simulink model "covid"  (R2019b)
settings: Solver=ode23s  StartTime=0.0  StopTime=50  FixedStep=1
values from neighbouring files (symbols this model uses):
  optimprob = optim.openProblem(Country, Province)    [main.m]
undefined symbols (not defined in the file or in its folder): D0, E0, I0, P0, Q0, R0, S0, x
settings Model: SimulationMode=accelerator  OrderedModelArguments=off  Creator=SaDiablo  LastModifiedBy=SaDiablo
settings SolverCC: MaxConsecutiveMinStep=1e4  ZeroCrossAlgorithm=Adaptive
settings DataIOCC: SaveState=on
settings DebuggingCC: MaxConsecutiveZCsMsg=warning  MaskedZcDiagnostic=none
settings HardwareCC: ProdHWDeviceType=AMD->x86-64 (Windows64)

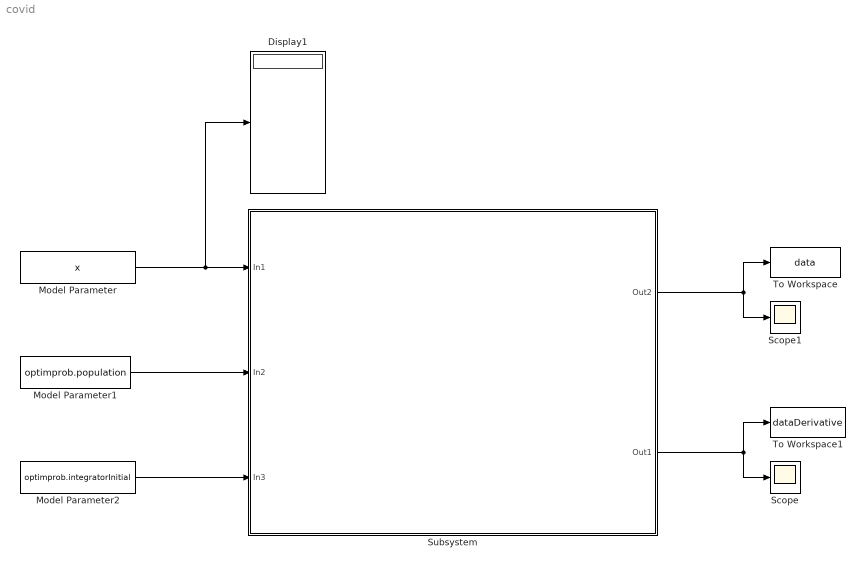
== system covid ==
  Display1 : Display
  Model Parameter : Constant  Value=x
  Model Parameter1 : Constant  Value=optimprob.population
  Model Parameter2 : Constant  Value=optimprob.integratorInitial
  Scope : Scope
  Scope1 : Scope
  Subsystem : Subsystem
  To Workspace : ToWorkspace  VariableName=data  SaveFormat=Timeseries  SampleTime=-1
  To Workspace1 : ToWorkspace  VariableName=dataDerivative  SaveFormat=Timeseries  SampleTime=-1
  wires:
  Model Parameter/1 -> Subsystem/1(In1), Display1/1
  Subsystem/1(Out2) -> Scope1/1, To Workspace/1
  Subsystem/2(Out1) -> Scope/1, To Workspace1/1
  Model Parameter2/1 -> Subsystem/3(In3)
  Model Parameter1/1 -> Subsystem/2(In2)

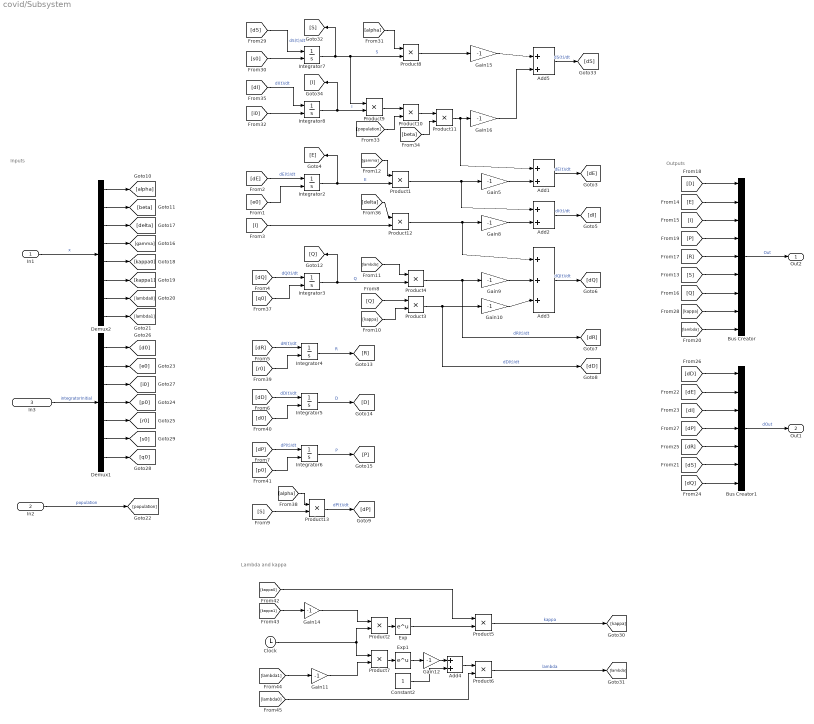
== system covid/Subsystem ==
  note: Inputs
  note: Outputs
  note: Lambda and kappa
  In1 : Inport
  In2 : Inport  Port=2
  In3 : Inport  Port=3
  Add1 : Sum  Inputs=+|+
  Add2 : Sum  Inputs=+|+
  Add3 : Sum  Inputs=+|+|+
  Add4 : Sum
  Add5 : Sum  Inputs=+|+
  Bus Creator : BusCreator  Inputs=9
  Bus Creator1 : BusCreator  Inputs=7
  Clock : Clock
  Constant2 : Constant
  Demux1 : Demux  Outputs=7
  Demux2 : Demux  Outputs=8
  Exp : Math  SignedPower=off  SaturateOnIntegerOverflow=on
  Exp1 : Math  SignedPower=off  SaturateOnIntegerOverflow=on
  Gain{5,8..12,14..16} (9 alike) : Gain  Gain=-1
  Integrator2 : Integrator  InitialConditionSource=external  InitialCondition=E0  LimitOutput=on  UpperSaturationLimit=optimprob.population  LowerSaturationLimit=0  WrappedStateUpperValue=population  WrappedStateLowerValue=0  ZeroCross=off  ContinuousStateAttributes='E'
  Integrator3 : Integrator  InitialConditionSource=external  InitialCondition=Q0  LimitOutput=on  UpperSaturationLimit=optimprob.population  LowerSaturationLimit=0  WrappedStateUpperValue=population  WrappedStateLowerValue=0  ZeroCross=off
  Integrator4 : Integrator  InitialConditionSource=external  InitialCondition=R0  LimitOutput=on  UpperSaturationLimit=optimprob.population  LowerSaturationLimit=0  WrappedStateUpperValue=population  WrappedStateLowerValue=0
  Integrator5 : Integrator  InitialConditionSource=external  InitialCondition=D0  LimitOutput=on  UpperSaturationLimit=optimprob.population  LowerSaturationLimit=0  WrappedStateUpperValue=population  WrappedStateLowerValue=0
  Integrator6 : Integrator  InitialConditionSource=external  InitialCondition=P0  LimitOutput=on  UpperSaturationLimit=optimprob.population  LowerSaturationLimit=0  WrappedStateUpperValue=population  WrappedStateLowerValue=0
  Integrator7 : Integrator  InitialConditionSource=external  InitialCondition=S0  LimitOutput=on  UpperSaturationLimit=optimprob.population  LowerSaturationLimit=0  WrappedStateUpperValue=population  WrappedStateLowerValue=0  ZeroCross=off
  Integrator8 : Integrator  InitialConditionSource=external  InitialCondition=I0  LimitOutput=on  UpperSaturationLimit=optimprob.population  LowerSaturationLimit=0  WrappedStateUpperValue=population  WrappedStateLowerValue=0  ZeroCross=off
  Product{1..13} (13 alike) : Product
  Out2 : Outport
  Out1 : Outport  Port=2
  wires:
  Integrator5/1 -> [D]  "D"
  Integrator4/1 -> [R]  "R"
  Integrator6/1 -> [P]  "P"
  [S] -> Product13/2
  [dR] -> Integrator4/1  "dR(t)/dt"
  [dP] -> Integrator6/1  "dP(t)/dt"
  [r0] -> Integrator4/2
  [d0] -> Integrator5/2
  [p0] -> Integrator6/2
  [dD] -> Integrator5/1  "dD(t)/dt"
  In1/1 -> Demux2/1  "x"
  Demux2/1 -> [alpha]
  Demux2/2 -> [beta]
  Demux2/8 -> [lambda1]
  Demux2/7 -> [lambda0]
  Demux2/6 -> [kappa1]
  Demux2/5 -> [kappa0]
  In2/1 -> [population]  "population"
  In3/1 -> Demux1/1  "integratorInitial"
  [lambda] -> Bus Creator/9
  [kappa] -> Bus Creator/8
  Bus Creator/1 -> Out2/1  "Out"
  Clock/1 -> Product7/1, Product2/2
  Product5/1 -> [kappa]  "kappa"
  Gain14/1 -> Product2/1
  Product2/1 -> Exp/1
  [kappa0] -> Product5/1
  [lambda1] -> Gain11/1
  Constant2/1 -> Add4/2
  Product6/1 -> [lambda]  "lambda"
  Product7/1 -> Exp1/1
  Gain12/1 -> Add4/1
  Exp1/1 -> Gain12/1
  [kappa1] -> Gain14/1
  Exp/1 -> Product5/2
  Bus Creator1/1 -> Out1/1  "dOut"
  [dS] -> Integrator7/1  "dS(t)/dt"
  [s0] -> Integrator7/2
  Integrator7/1 -> Product9/1, Product8/2, [S]  "S"
  [alpha] -> Product8/1
  Product8/1 -> Gain15/1
  Gain15/1 -> Add5/1
  Product9/1 -> Product10/1
  [population] -> Product10/2
  Product10/1 -> Product11/1
  [beta] -> Product11/2
  Gain16/1 -> Add5/2
  Add5/1 -> [dS]  "dS(t)/dt"
  [dI] -> Integrator8/1  "dI(t)/dt"
  [i0] -> Integrator8/2
  Integrator8/1 -> [I], Product9/2  "I"
  [I] -> Product12/2
  Gain10/1 -> Add3/3
  Product3/1 -> [dD], Gain10/1  "dD(t)/dt"
  [e0] -> Integrator2/2
  Add2/1 -> [dI]  "dI(t)/dt"
  [kappa] -> Product3/2
  [Q] -> Product3/1
  Integrator3/1 -> Product4/2, [Q]  "Q"
  Product12/1 -> Add3/1, Gain8/1
  Add3/1 -> [dQ]  "dQ(t)/dt"
  [dQ] -> Integrator3/1  "dQ(t)/dt"
  Gain5/1 -> Add1/2
  Product4/1 -> [dR], Gain9/1  "dR(t)/dt"
  Integrator2/1 -> [E], Product1/2  "E"
  Add1/1 -> [dE]  "dE(t)/dt"
  [dE] -> Integrator2/1  "dE(t)/dt"
  Product11/1 -> Add1/1, Gain16/1
  [lambda] -> Product4/1
  Gain9/1 -> Add3/2
  Gain8/1 -> Add2/2
  Product1/1 -> Add2/1, Gain5/1
  [gamma] -> Product1/1
  [delta] -> Product12/1
  [q0] -> Integrator3/2
  [alpha] -> Product13/1
  Product13/1 -> [dP]  "dP(t)/dt"
  Gain11/1 -> Product7/2
  Add4/1 -> Product6/1
  [lambda0] -> Product6/2
  Demux1/1 -> [d0]
  Demux1/7 -> [q0]
  Demux1/2 -> [e0]
  Demux1/3 -> [i0]
  Demux1/4 -> [p0]
  Demux1/5 -> [r0]
  Demux1/6 -> [s0]
  Demux2/3 -> [delta]
  Demux2/4 -> [gamma]
  [D] -> Bus Creator/1
  [E] -> Bus Creator/2
  [I] -> Bus Creator/3
  [P] -> Bus Creator/4
  [R] -> Bus Creator/5
  [S] -> Bus Creator/6
  [Q] -> Bus Creator/7
  [dD] -> Bus Creator1/1
  [dQ] -> Bus Creator1/7
  [dE] -> Bus Creator1/2
  [dI] -> Bus Creator1/3
  [dP] -> Bus Creator1/4
  [dR] -> Bus Creator1/5
  [dS] -> Bus Creator1/6
